simulink model "Dubug_model"  (R2014a)
settings: Solver=ode45  StartTime=0.0  StopTime=1000  MaxStep=0.1  RelTol=1e-9
values from neighbouring files (symbols this model uses):
  I = diag([Ixx;Iyy;Izz])    [Satellite_Setup_Sun_Pointing (1).m]    (also in Satellite_Setup_Sun_Pointing.m; Satellite_setup_ZenithPointing (1).m; Satellite_setup_ZenithPointing.m)
  kd = 6e-4    (= 0.0006)    [Example__simulaltion (1).m]    (also in Example__simulaltion.m; PD_SunPoint_setup (1).m = 2; PD_zenith_setup (1).m = 0.0002; PD_zenith_setup.m = 0.0002)
  kp = 5e-9    (= 5e-09)    [Example__simulaltion (1).m]    (also in Example__simulaltion.m; PD_SunPoint_setup (1).m = 0.0006; PD_zenith_setup (1).m = 1.6e-07; PD_zenith_setup.m = 1.6e-07)
  omega_orbit = [0;-7.67/(401.1+6371);0]    [Satellite_Setup_Sun_Pointing (1).m]    (also in Satellite_Setup_Sun_Pointing.m; Satellite_setup_ZenithPointing (1).m; Satellite_setup_ZenithPointing.m)
  q_ref = q_3_ref    [Example__simulaltion (1).m]    (also in Example__simulaltion.m)
  x_0 = transpose([wb_bi_init,qb_i_init])    [Example__simulaltion (1).m]    (also in Example__simulaltion.m; Satellite_Setup_Sun_Pointing (1).m = [transpose(wb_bi_init),qb_i_init]; Satellite_Setup_Sun_Pointing.m = [transpose(wb_bi_init),qb_i_init]; Satellite_setup_ZenithPointing (1).m = [(wb_bi_init),qb_i_init])
  x_orbit_init = [long_init,lat_init,altitude,qb_o_init,qo_i_init]    [Example__simulaltion (1).m]    (also in Example__simulaltion.m; Satellite_Setup_Sun_Pointing (1).m; Satellite_Setup_Sun_Pointing.m; Satellite_setup_ZenithPointing (1).m)
undefined symbols (not defined in the file or in its folder): SkewSym
libraries: aerolibtransform2 x4, vrlib x3
settings Model: Creator=Daire  LastModifiedBy=Daire

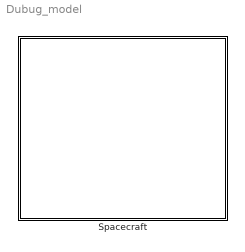
== system Dubug_model ==
  Spacecraft : Subsystem  VariantControl=Variant1

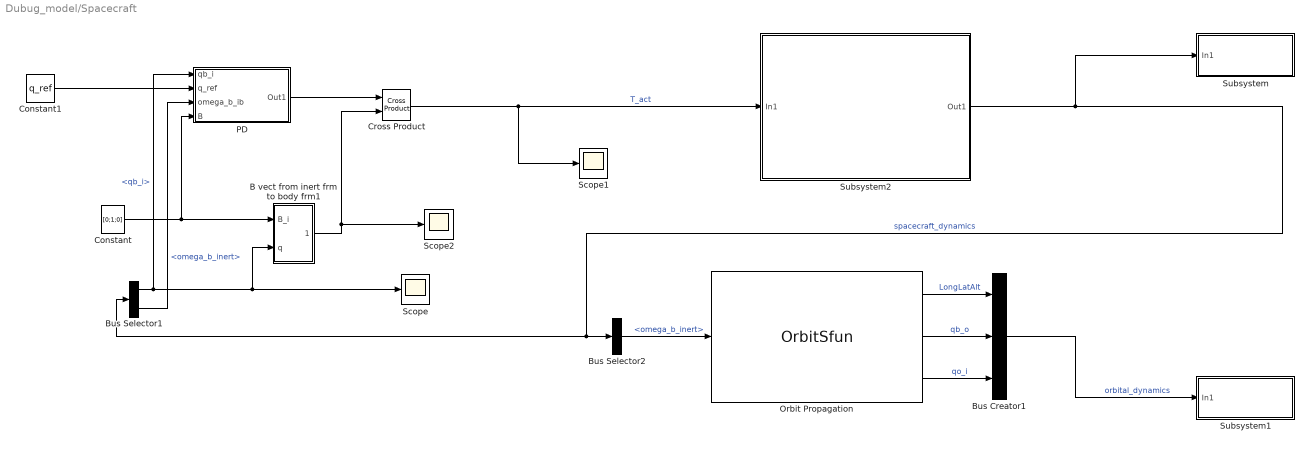
== system Dubug_model/Spacecraft ==
  B vect from inert frm to body frm1 : Subsystem
  Bus Creator1 : BusCreator  Inputs=3
  Bus Selector1 : BusSelector  OutputSignals=qb_i,omega_b_inert
  Bus Selector2 : BusSelector  OutputSignals=omega_b_inert
  Constant : Constant  Value=[0;1;0]
  Constant1 : Constant  Value=q_ref
  Cross Product : vrlib/Utilities/Cross Product
  Orbit Propagation : M-S-Function  FunctionName=OrbitSfun  Parameters=x_orbit_init,omega_orbit  mask{Parameter1=x_orbit_init, Parameter2=omega_orbit}
      mask prompts: Parameter1 "Initial orbit param"; Parameter2 "orbit angular velocity"
      mask DialogControl Control8 Prompt: Orbit properties
      mask Display:
      | disp('Orbital Parameters')
      | port_label('input',1,'ang vel')
      | port_label('output',1,'LLA')
      | port_label('output',2,'qb_o')
      | port_label('output',3,'qo_i')
  PD : Subsystem  TreatAsAtomicUnit=on
  Scope : Scope
  Scope1 : Scope
  Scope2 : Scope
      settings: YMin=-0.5  YMax=2.5  SaveName=ScopeData2
  Subsystem : Subsystem
  Subsystem1 : Subsystem
  Subsystem2 : Subsystem  VariantControl=(default)
  wires:
  Bus Selector2/1 -> Orbit Propagation/1  "<omega_b_inert>"
  Subsystem2/1(Out1) -> Subsystem/1(In1), Bus Selector2/1, Bus Selector1/1  "spacecraft_dynamics"
  Bus Creator1/1 -> Subsystem1/1(In1)  "orbital_dynamics"
  Orbit Propagation/1 -> Bus Creator1/1  "LongLatAlt"
  Orbit Propagation/2 -> Bus Creator1/2  "qb_o"
  Orbit Propagation/3 -> Bus Creator1/3  "qo_i"
  Cross Product/1 -> Scope1/1, Subsystem2/1(In1)  "T_act"
  PD/1(Out1) -> Cross Product/1
  Bus Selector1/1 -> PD/1(qb_i), B vect from inert frm to body frm1/2(q), Scope/1  "<qb_i>"
  B vect from inert frm to body frm1/1(B_b) -> Scope2/1, Cross Product/2
  Constant/1 -> B vect from inert frm to body frm1/1(B_i), PD/4(B)
  Bus Selector1/2 -> PD/3(omega_b_ib)  "<omega_b_inert>"
  Constant1/1 -> PD/2(q_ref)

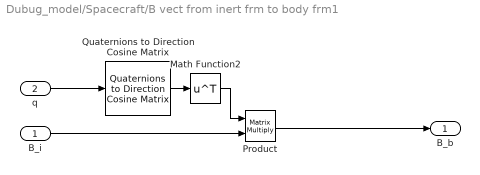
== system Dubug_model/Spacecraft/B vect from inert frm to body frm1 ==
  B_i : Inport
  q : Inport  Port=2
  Math Function2 : Math  Operator=transpose  SaturateOnIntegerOverflow=on
  Product : Product  Multiplication=Matrix(*)
  Quaternions to Direction Cosine Matrix : aerolibtransform2/Quaternions to  Direction Cosine Matrix
  B_b : Outport
  wires:
  B_i/1 -> Product/2
  Product/1 -> B_b/1
  Math Function2/1 -> Product/1
  q/1 -> Quaternions to Direction Cosine Matrix/1
  Quaternions to Direction Cosine Matrix/1 -> Math Function2/1

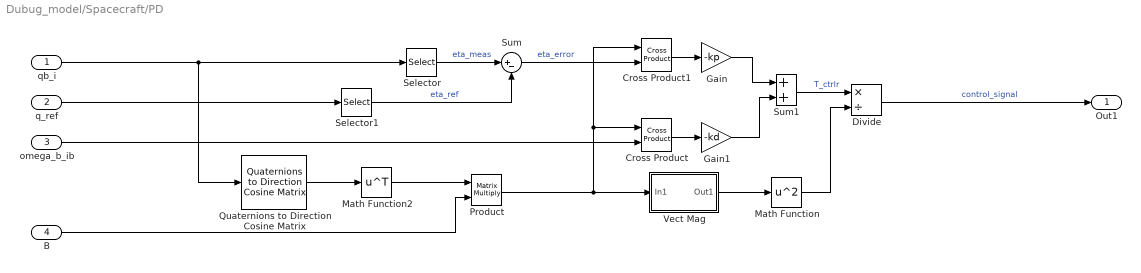
== system Dubug_model/Spacecraft/PD ==
  qb_i : Inport
  q_ref : Inport  Port=2
  omega_b_ib : Inport  Port=3
  B : Inport  Port=4
  Cross Product : vrlib/Utilities/Cross Product
  Cross Product1 : vrlib/Utilities/Cross Product
  Divide : Product  Inputs=*/
  Gain : Gain  Gain=-kp
  Gain1 : Gain  Gain=-kd
  Math Function : Math  Operator=square  SaturateOnIntegerOverflow=on
  Math Function2 : Math  Operator=transpose  SaturateOnIntegerOverflow=on
  Product : Product  Multiplication=Matrix(*)
  Quaternions to Direction Cosine Matrix : aerolibtransform2/Quaternions to  Direction Cosine Matrix
  Selector : Selector  InputPortWidth=4  Indices=[2 3 4]
  Selector1 : Selector  InputPortWidth=4  Indices=[2 3 4]
  Sum : Sum  Inputs=|+-
  Sum1 : Sum
  Vect Mag : Subsystem
  Out1 : Outport
  wires:
  Selector/1 -> Sum/1  "eta_meas"
  Cross Product1/1 -> Gain/1
  Vect Mag/1(Out1) -> Math Function/1
  Math Function2/1 -> Product/1
  Selector1/1 -> Sum/2  "eta_ref"
  Sum1/1 -> Divide/1  "T_ctrlr"
  omega_b_ib/1 -> Cross Product/2
  qb_i/1 -> Quaternions to Direction Cosine Matrix/1, Selector/1
  Sum/1 -> Cross Product1/2  "eta_error"
  Gain/1 -> Sum1/1
  Product/1 -> Cross Product1/1, Cross Product/1, Vect Mag/1(In1)
  Gain1/1 -> Sum1/2
  Quaternions to Direction Cosine Matrix/1 -> Math Function2/1
  Divide/1 -> Out1/1  "control_signal"
  B/1 -> Product/2
  q_ref/1 -> Selector1/1
  Cross Product/1 -> Gain1/1
  Math Function/1 -> Divide/2

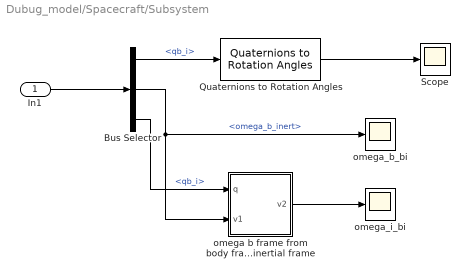
== system Dubug_model/Spacecraft/Subsystem ==
  In1 : Inport
  Bus Selector : BusSelector  OutputSignals=qb_i,omega_b_inert,qb_i
  Quaternions to Rotation Angles : aerolibtransform2/Quaternions to Rotation Angles  rotationOrder=XYZ
  Scope : Scope
      settings: TimeRange=10  YMin=-3.5  YMax=3.5  SaveName=ScopeData5
  omega b frame from body frame comp to inertial frame : Subsystem
  omega_b_bi : Scope
      settings: TimeRange=10  YMin=-700  YMax=0  SaveName=ScopeData6
  omega_i_bi : Scope
      settings: YMin=-0.0025  YMax=0.0025  SaveName=ScopeData18
  wires:
  In1/1 -> Bus Selector/1
  Bus Selector/1 -> Quaternions to Rotation Angles/1  "<qb_i>"
  Quaternions to Rotation Angles/1 -> Scope/1
  Bus Selector/2 -> omega b frame from body frame comp to inertial frame/2(v1), omega_b_bi/1  "<omega_b_inert>"
  Bus Selector/3 -> omega b frame from body frame comp to inertial frame/1(q)  "<qb_i>"
  omega b frame from body frame comp to inertial frame/1(v2) -> omega_i_bi/1

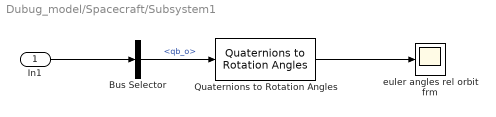
== system Dubug_model/Spacecraft/Subsystem1 ==
  In1 : Inport
  Bus Selector : BusSelector  OutputSignals=qb_o
  Quaternions to Rotation Angles : aerolibtransform2/Quaternions to Rotation Angles  rotationOrder=XYZ
  euler angles rel orbit frm : Scope
      settings: TimeRange=22000  YMin=-0.7  YMax=0.9  SaveName=ScopeData5
  wires:
  Quaternions to Rotation Angles/1 -> euler angles rel orbit frm/1
  Bus Selector/1 -> Quaternions to Rotation Angles/1  "<qb_o>"
  In1/1 -> Bus Selector/1

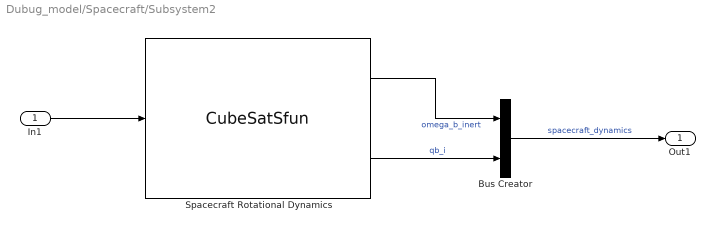
== system Dubug_model/Spacecraft/Subsystem2 ==
  In1 : Inport
  Bus Creator : BusCreator  Inputs=2
  Spacecraft Rotational Dynamics : M-S-Function  FunctionName=CubeSatSfun  Parameters=x_0,I  mask{Parameter2=x_0, Parameter3=I}
      mask prompts: Parameter2 "x_0"; Parameter3 "I"
      mask DialogControl DescTextVar Prompt: Model of a rigid CubeSat. Model takes Torque about each axis as an input. The first output is the angular velocity of the sat wrt an inertial frame. The second output is the quaternion which represents the rotation between inertial and body fixed frames
      mask Display:
      | disp('Cube Sat Model')
      | port_label('input',1,'Torq')
      | port_label('output',1,'Ang Vel')
      | port_label('output',2,'Quat')
  Out1 : Outport
  wires:
  Bus Creator/1 -> Out1/1  "spacecraft_dynamics"
  In1/1 -> Spacecraft Rotational Dynamics/1
  Spacecraft Rotational Dynamics/1 -> Bus Creator/1  "omega_b_inert"
  Spacecraft Rotational Dynamics/2 -> Bus Creator/2  "qb_i"

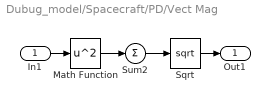
== system Dubug_model/Spacecraft/PD/Vect Mag ==
  In1 : Inport
  Math Function : Math  Operator=square  SaturateOnIntegerOverflow=on
  Sqrt : Sqrt  SaturateOnIntegerOverflow=on
  Sum2 : Sum  Inputs=+
  Out1 : Outport
  wires:
  Sqrt/1 -> Out1/1
  In1/1 -> Math Function/1
  Math Function/1 -> Sum2/1
  Sum2/1 -> Sqrt/1

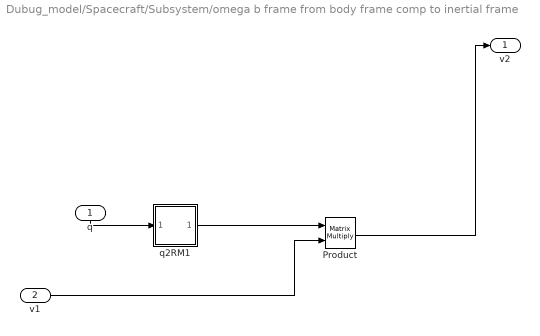
== system Dubug_model/Spacecraft/Subsystem/omega b frame from body frame comp to inertial frame ==
  q : Inport
  v1 : Inport  Port=2
  Product : Product  Multiplication=Matrix(*)
  q2RM1 : Subsystem
  v2 : Outport
  wires:
  q/1 -> q2RM1/1(In1)
  q2RM1/1(Out1) -> Product/1
  v1/1 -> Product/2
  Product/1 -> v2/1

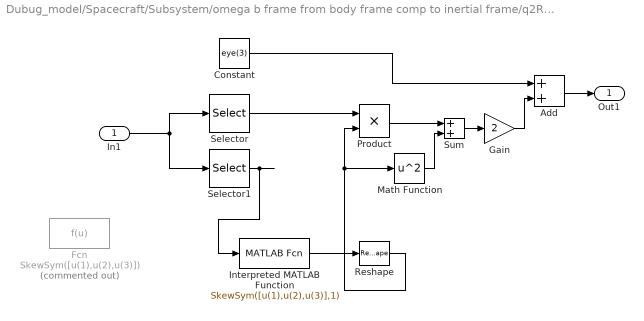
== system Dubug_model/Spacecraft/Subsystem/omega b frame from body frame comp to inertial frame/q2RM1 ==
  In1 : Inport
  Add : Sum
  Constant : Constant  Value=eye(3)
  Fcn : Fcn  Commented=on  Expr=SkewSym([u(1),u(2),u(3)])
  Gain : Gain  Gain=2
  Interpreted MATLAB Function : MATLABFcn  MATLABFcn=SkewSym([u(1),u(2),u(3)],1)  OutputDimensions=9
  Math Function : Math  Operator=square  SaturateOnIntegerOverflow=on
  Product : Product
  Reshape : Reshape  OutputDimensionality=Customize  OutputDimensions=[3,3]
  Selector : Selector  InputPortWidth=4  Indices=[1]
  Selector1 : Selector  InputPortWidth=4  Indices=[2 3 4]
  Sum : Sum
  Out1 : Outport
  wires:
  Interpreted MATLAB Function/1 -> Reshape/1
  Add/1 -> Out1/1
  Constant/1 -> Add/1
  Gain/1 -> Add/2
  Sum/1 -> Gain/1
  Math Function/1 -> Sum/2
  Product/1 -> Sum/1
  Selector1/1 -> Interpreted MATLAB Function/1
  Selector/1 -> Product/1
  Reshape/1 -> Product/2, Math Function/1
  In1/1 -> Selector1/1, Selector/1
